simulink model "lanedetection"  (R2018a)
settings: Solver=FixedStepAuto  StartTime=0.0  StopTime=inf  RelTol=1e-3  EnableMultiTasking=on
libraries: visiongeotforms x3, embdlinuxlib x2, raspberrypilib x1
settings Model: SimulationMode=external  Creator=ifadmin  LastModifiedBy=ifadmin
settings SolverCC: PositivePriorityOrder=on
settings OptimizationCC: EnhancedBackFolding=on  PassReuseOutputArgsAs=Individual arguments  MaxStackSize=64  OptimizeBlockOrder=speed  DifferentSizesBufferReuse=on  OptimizationCustomize=off
settings DebuggingCC: ParameterTunabilityLossMsg=error
settings HardwareCC: ProdBitPerPointer=32  ProdBitPerSizeT=32  ProdBitPerPtrDiffT=32  ProdLargestAtomicInteger=Long  ProdLargestAtomicFloat=Double  ProdWordSize=32  ProdHWDeviceType=ARM Compatible->ARM Cortex
settings SFSimCC: MATLABDynamicMemAlloc=off
settings RTWCC: SystemTargetFile=ert.tlc  HardwareBoard=Raspberry Pi  TLCOptions="-aInlineSetEventsForThisBaseRateFcn=TLC_FALSE -aSuppressMultiTaskScheduler=TLC_FALSE  -aRateBasedStepFcn=0"  TemplateMakefile=ert_default_tmf  GenerateReport=on  Toolchain=GNU GCC Raspberry Pi  BuildConfiguration=Faster Runs  IncludeHyperlinkInReport=on  LaunchReport=on  GenerateTraceInfo=on  GenerateTraceReport=on  GenerateTraceReportSl=on  GenerateTraceReportSf=on  GenerateTraceReportEml=on
settings CodeAppCC: ForceParamTrailComments=on  IgnoreCustomStorageClasses=off  OperatorAnnotations=on  SimulinkDataObjDesc=on  SFDataObjDesc=on  InsertBlockDesc=on
settings ERTTargetCC: SupportVariableSizeSignals=on

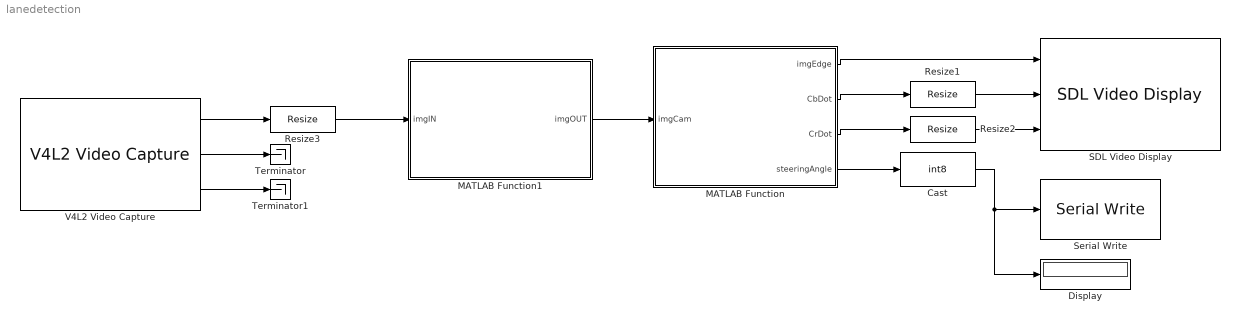
== system lanedetection ==
  Cast : DataTypeConversion  OutDataTypeStr=int8  ConvertRealWorld=Stored Integer (SI)  LockScale=on
  Display : Display
      settings: Format=decimal (Stored Integer)
  MATLAB Function : MATLAB Function  TreatAsAtomicUnit=on
  MATLAB Function1 : MATLAB Function  TreatAsAtomicUnit=on
  Resize1 : visiongeotforms/Resize  specify=Output size as a percentage of input size  rfactor=[50 100]  outCols=25  outRows=25  outRowsCols=[25 35]  interp_method=Bilinear  antialias=on  useROI=off  roiFlag=off  prodOutputMode=Binary point scaling  prodOutputWordLength=32  prodOutputFracLength=10  roundingMode=Nearest  overflowMode=on
      settings: SourceProductName=Computer Vision System Toolbox  SourceProductBaseCode=VP
  Resize2 : visiongeotforms/Resize  specify=Output size as a percentage of input size  rfactor=[50 100]  outCols=25  outRows=25  outRowsCols=[25 35]  interp_method=Bilinear  antialias=on  useROI=off  roiFlag=off  prodOutputMode=Binary point scaling  prodOutputWordLength=32  prodOutputFracLength=10  roundingMode=Nearest  overflowMode=on
      settings: SourceProductName=Computer Vision System Toolbox  SourceProductBaseCode=VP
  Resize3 : visiongeotforms/Resize  specify=Output size as a percentage of input size  rfactor=[20 20]  outCols=25  outRows=25  outRowsCols=[25 35]  interp_method=Bilinear  antialias=on  useROI=off  roiFlag=off  prodOutputMode=Binary point scaling  prodOutputWordLength=32  prodOutputFracLength=10  roundingMode=Nearest  overflowMode=on
      settings: SourceProductName=Computer Vision System Toolbox  SourceProductBaseCode=VP
  SDL Video Display : embdlinuxlib/SDL Video Display  pixelFormat=YCbCr 4:2:2  pixelOrder=Planar  rowMajor=on  blockPlatform=Raspberry Pi
      settings: SourceProductName=Simulink Support Package for Raspberry Pi Hardware  SourceProductBaseCode=RASPPI
  Serial Write : raspberrypilib/Serial Write  board=Pi 3 Model B  SCIModule_=/dev/ttyACM0  Baudrate_=9600  Parity=None  StopBits_=1  HardwareFlowControl=None  ByteOrder=LittleEndian  OutputStatus=off  blockPlatform=RaspberryPi
      settings: SourceProductName=Simulink Support Package for Raspberry Pi Hardware  SourceProductBaseCode=RASPPI
  Terminator : Terminator
  Terminator1 : Terminator
  V4L2 Video Capture : embdlinuxlib/V4L2 Video Capture  m_devName='/dev/video0'  roi=[0, 0, 640, 480]  imSizeSelection=800x600  imSize=[640, 480]  pixelFormat=YCbCr 4:2:2  pixelOrder=Planar  sampleTime=1/20  simOutput=Colorbars  blockPlatform=Raspberry Pi
      settings: SourceProductName=Simulink Support Package for Raspberry Pi Hardware  SourceProductBaseCode=RASPPI
  wires:
  MATLAB Function/1(imgEdge) -> SDL Video Display/1
  MATLAB Function/2(CbDot) -> Resize1/1
  MATLAB Function/3(CrDot) -> Resize2/1
  Resize1/1 -> SDL Video Display/2
  Resize2/1 -> SDL Video Display/3
  V4L2 Video Capture/1 -> Resize3/1
  V4L2 Video Capture/2 -> Terminator/1
  V4L2 Video Capture/3 -> Terminator1/1
  MATLAB Function1/1(imgOUT) -> MATLAB Function/1("imgCam ")
  Resize3/1 -> MATLAB Function1/1(imgIN)
  MATLAB Function/4(steeringAngle) -> Cast/1
  Cast/1 -> Display/1, Serial Write/1

== matlab function lanedetection/MATLAB Function1 ==
  data: imgIN input uint8 size=[160 120]; imgOUT output uint8 size=[160 30]
function imgOUT   = imgROI(imgIN)

    % imgIN Array von 160x120
    % rectangle('Position',[x,y,w,h])
    
    imgOUT = imgIN(1:160,66:95);

end

== matlab function lanedetection/MATLAB Function ==
  data: imgCam input size=[160 30]; imgEdge output size=[160 30]; CbDot output size=[160 30]; CrDot output size=[160 30]; steeringAngle output
function [imgEdge, CbDot, CrDot,  steeringAngle]  = lanedetection(imgCam)

    threshold = 40;
    
    % convert to grayscale
    % imgGray = rgb2gray(imgCam);

    % create laplacian filter
    k = [1 2 1; 0 0 0; -1 -2 -1];
    % run sobel
    V = conv2(double(imgCam),k','same');
    
    % filter edges
    imgEdges = uint8((V > threshold) * 255);
    
    % coordinates of all detected objects
    [x, y] = find(imgEdges);
    
    % detect the center of all objects
    xCenter = round(mean(x));
    yCenter = round(mean(y));
    
    % create vector xx and yy for an area around the center of all objects
    xx = max(1, xCenter-2):min(xCenter+2, size(imgEdges, 1));
    yy = max(1, yCenter-2):min(yCenter+2, size(imgEdges, 2));
    
    % create new array with the size of "bw" and fill it with "0"
    bwdot = zeros(size(imgEdges), 'uint8');
    
    % if there is something detected at x and y...
    if ~isempty(x) && ~isempty(y)
        % ...mark the area around the center
        bwdot(xx, yy) = 255;
    % if nothing gets detected...
    else
        bwdot(xx, yy) = 0;
    end
    
    % add the marked area around the center to the array justRed
    imgEdge = imgEdges + bwdot;
    CbDot = bwdot;
    CrDot = bwdot;
    steeringAngle = (xCenter - 80);
end
